simulink library "dynamics_lib"  (R2023b)
settings: Solver=VariableStepAuto  StartTime=0.0  StopTime=10.0  RelTol=1e-3
libraries: Raptor_lib x129, cstblocks x1, autolibshared x1
(part 1 of 2)
settings Model: Creator=serga  LastModifiedBy=serga
settings OptimizationCC: ReuseModelBlockBuffer=off

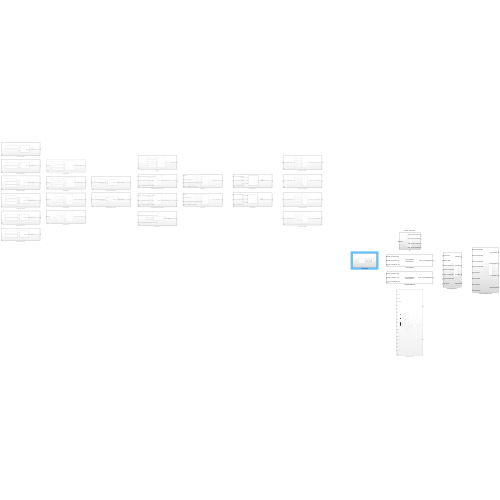
[thumbnail: Simulink's stored preview of the top-level diagram]
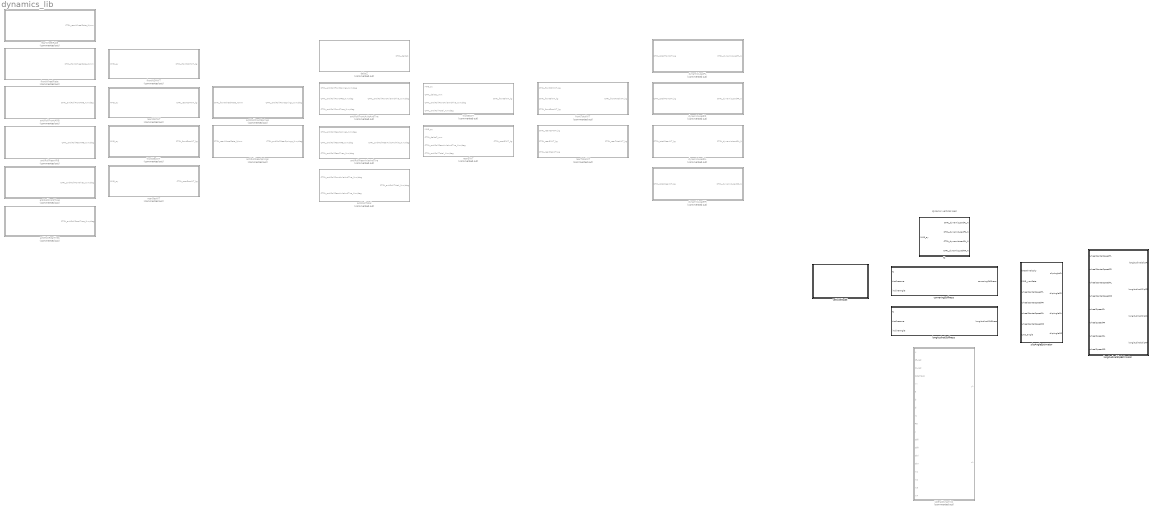
== system dynamics_lib ==
  note: dynamic vertical load
  antiRollFrontARB : Subsystem  Commented=on  TreatAsAtomicUnit=on
  antiRollFrontAxleAndTire : Subsystem  Commented=on  TreatAsAtomicUnit=on
  antiRollFrontSprings : Subsystem  Commented=on  TreatAsAtomicUnit=on
  antiRollFrontTires : Subsystem  Commented=on  TreatAsAtomicUnit=on
  antiRollRearARB : Subsystem  Commented=on  TreatAsAtomicUnit=on
  antiRollRearAxleAndTire : Subsystem  Commented=on  TreatAsAtomicUnit=on
  antiRollRearSprings : Subsystem  Commented=on  TreatAsAtomicUnit=on
  antiRollRearTires : Subsystem  Commented=on  TreatAsAtomicUnit=on
  antiRollTotal : Subsystem  Commented=on  TreatAsAtomicUnit=on
  corneringStiffness : Subsystem  mask{pos=''}
      mask Display:
      | disp(['corneringStiffness\n'...
      |     'Wheel Position: ' pos]);
      | port_label('input', 1, ['CTRL_dynamicLoad' pos '_N']);
      | port_label('input', 2, ['CTRL_tirePressure' pos '_bar']);
      | port_label('input', 3, ['CTRL_inclineAngle' pos '_deg']);
      | port_label('output', 1, ['CTRL_corneringStiffness' pos]);
  deltaZ : Subsystem  Commented=on  TreatAsAtomicUnit=on
  dynamicLoadFL : Subsystem  Commented=on  TreatAsAtomicUnit=on
  dynamicLoadFR : Subsystem  Commented=on  TreatAsAtomicUnit=on
  dynamicLoadRL : Subsystem  Commented=on  TreatAsAtomicUnit=on
  dynamicLoadRR : Subsystem  Commented=on  TreatAsAtomicUnit=on
  frontElWT : Subsystem  Commented=on  TreatAsAtomicUnit=on
  frontGeoWT : Subsystem  Commented=on  TreatAsAtomicUnit=on
  frontNSMWT : Subsystem  Commented=on
  frontTotalWT : Subsystem  Commented=on  TreatAsAtomicUnit=on
  frontWheelRate : Subsystem  Commented=on  TreatAsAtomicUnit=on
  fz : Subsystem
  lateralDynamics : Subsystem  Commented=on
  longitudinalSlipEstimator : Subsystem
  longitudinalStiffness : Subsystem  mask{pos=''}
      mask Display:
      | disp(['longitudinalStiffness\n'...
      |     'Wheel Position: ' pos]);
      | port_label('input', 1, ['CTRL_dynamicLoad' pos '_N']);
      | port_label('input', 2, ['CTRL_tirePressure' pos '_bar']);
      | port_label('input', 3, ['CTRL_inclineAngle' pos '_deg']);
      | port_label('output', 1, ['CTRL_longitudinalStiffness' pos]);
  rearElWT : Subsystem  Commented=on  TreatAsAtomicUnit=on
  rearGeoWT : Subsystem  Commented=on  TreatAsAtomicUnit=on
  rearNSMWT : Subsystem  Commented=on  TreatAsAtomicUnit=on
  rearTotalWT : Subsystem  Commented=on  TreatAsAtomicUnit=on
  rearWheelRate : Subsystem  Commented=on  TreatAsAtomicUnit=on
  slipAngleEstimator : Subsystem
  vehicleModel : Subsystem

== system dynamics_lib/antiRollFrontARB ==
  antiRollFrontARB : MATLAB Function  TreatAsAtomicUnit=on
  raptor_data_read : Raptor_lib/Data Storage/raptor_data_read  dataName='DATA_frontTrack_mm'  dataShape=Scalar  idxSource=Input  idxRow=1  idxCol=1
      settings: SourceProductName=Raptor
  raptor_data_read1 : Raptor_lib/Data Storage/raptor_data_read  dataName='DATA_frontARBStiffness_Npmm'  dataShape=Scalar  idxSource=Input  idxRow=1  idxCol=1
      settings: SourceProductName=Raptor
  raptor_data_read2 : Raptor_lib/Data Storage/raptor_data_read  dataName='DATA_frontARBMotionRatio_mmpmm'  dataShape=Scalar  idxSource=Input  idxRow=1  idxCol=1
      settings: SourceProductName=Raptor
  CTRL_antiRollFrontARB_N.m/deg : Outport
  wires:
  antiRollFrontARB/1(antiRollFrontARB) -> CTRL_antiRollFrontARB_N.m/deg/1
  raptor_data_read2/1 -> antiRollFrontARB/3(frontARBMotionRatio)
  raptor_data_read1/1 -> antiRollFrontARB/1(frontARBStiffness)
  raptor_data_read/1 -> antiRollFrontARB/2(frontTrack)

== system dynamics_lib/antiRollFrontAxleAndTire ==
  CTRL_antiRollFrontSprings_N.m/deg : Inport
  CTRL_antiRollFrontARB_N.m/deg : Inport  Port=2
  CTRL_antiRollFrontTires_N.m/deg : Inport  Port=3
  antiRollFrontAxleAndTire : MATLAB Function  TreatAsAtomicUnit=on
  CTRL_antiRollFrontAxleAndTire_N.m/deg : Outport
  wires:
  CTRL_antiRollFrontSprings_N.m/deg/1 -> antiRollFrontAxleAndTire/1(antiRollFrontSprings)
  CTRL_antiRollFrontARB_N.m/deg/1 -> antiRollFrontAxleAndTire/2(antiRollFrontARB)
  CTRL_antiRollFrontTires_N.m/deg/1 -> antiRollFrontAxleAndTire/3(antiRollFrontTires)
  antiRollFrontAxleAndTire/1(antiRollFrontAxleAndTire) -> CTRL_antiRollFrontAxleAndTire_N.m/deg/1

== system dynamics_lib/antiRollFrontSprings ==
  CTRL_frontWheelRate_N/mm : Inport
  antiRollFrontSprings : MATLAB Function  TreatAsAtomicUnit=on
  raptor_data_read : Raptor_lib/Data Storage/raptor_data_read  dataName='DATA_frontTrack_mm'  dataShape=Scalar  idxSource=Input  idxRow=1  idxCol=1
      settings: SourceProductName=Raptor
  CTRL_antiRollFrontSprings_N.m/deg : Outport
  wires:
  raptor_data_read/1 -> antiRollFrontSprings/1(frontTrack)
  CTRL_frontWheelRate_N/mm/1 -> antiRollFrontSprings/2(frontWheelRate)
  antiRollFrontSprings/1(antiRollFrontSprings) -> CTRL_antiRollFrontSprings_N.m/deg/1

== system dynamics_lib/antiRollFrontTires ==
  antiRollFrontTires : MATLAB Function  TreatAsAtomicUnit=on
  raptor_data_read : Raptor_lib/Data Storage/raptor_data_read  dataName='DATA_frontTrack_mm'  dataShape=Scalar  idxSource=Input  idxRow=1  idxCol=1
      settings: SourceProductName=Raptor
  raptor_data_read1 : Raptor_lib/Data Storage/raptor_data_read  dataName='DATA_frontTireStiffness_Npmm'  dataShape=Scalar  idxSource=Input  idxRow=1  idxCol=1
      settings: SourceProductName=Raptor
  CTRL_antiRollFrontTires_N.m/deg : Outport
  wires:
  raptor_data_read1/1 -> antiRollFrontTires/2(frontTireStiffness)
  raptor_data_read/1 -> antiRollFrontTires/1(frontTrack)
  antiRollFrontTires/1(antiRollFrontTires) -> CTRL_antiRollFrontTires_N.m/deg/1

== system dynamics_lib/antiRollRearARB ==
  antiRollRearARB : MATLAB Function  TreatAsAtomicUnit=on
  raptor_data_read : Raptor_lib/Data Storage/raptor_data_read  dataName='DATA_rearTrack_mm'  dataShape=Scalar  idxSource=Input  idxRow=1  idxCol=1
      settings: SourceProductName=Raptor
  raptor_data_read1 : Raptor_lib/Data Storage/raptor_data_read  dataName='DATA_rearARBStiffness_Npmm'  dataShape=Scalar  idxSource=Input  idxRow=1  idxCol=1
      settings: SourceProductName=Raptor
  raptor_data_read2 : Raptor_lib/Data Storage/raptor_data_read  dataName='DATA_rearARBMotionRatio_mmpmm'  dataShape=Scalar  idxSource=Input  idxRow=1  idxCol=1
      settings: SourceProductName=Raptor
  CTRL_antiRollRearARB_N.m/deg : Outport
  wires:
  raptor_data_read2/1 -> antiRollRearARB/3(rearARBMotionRatio)
  raptor_data_read1/1 -> antiRollRearARB/1(rearARBStiffness)
  raptor_data_read/1 -> antiRollRearARB/2(rearTrack)
  antiRollRearARB/1(antiRollRearARB) -> CTRL_antiRollRearARB_N.m/deg/1

== system dynamics_lib/antiRollRearAxleAndTire ==
  CTRL_antiRollRearSprings_N.m/deg : Inport
  CTRL_antiRollRearARB_N.m/deg : Inport  Port=2
  CTRL_antiRollRearTires_N.m/deg : Inport  Port=3
  antiRollRearAxleAndTire : MATLAB Function  TreatAsAtomicUnit=on
  CTRL_antiRollRearAxleAndTire_N.m/deg : Outport
  wires:
  CTRL_antiRollRearSprings_N.m/deg/1 -> antiRollRearAxleAndTire/1(antiRollRearSprings)
  CTRL_antiRollRearARB_N.m/deg/1 -> antiRollRearAxleAndTire/2(antiRollRearARB)
  CTRL_antiRollRearTires_N.m/deg/1 -> antiRollRearAxleAndTire/3(antiRollRearTires)
  antiRollRearAxleAndTire/1(antiRollRearAxleAndTire) -> CTRL_antiRollRearAxleAndTire_N.m/deg/1

== system dynamics_lib/antiRollRearSprings ==
  CTRL_rearWheelRate_N/mm : Inport
  antiRollRearSprings : MATLAB Function  TreatAsAtomicUnit=on
  raptor_data_read : Raptor_lib/Data Storage/raptor_data_read  dataName='DATA_rearTrack_mm'  dataShape=Scalar  idxSource=Input  idxRow=1  idxCol=1
      settings: SourceProductName=Raptor
  CTRL_antiRollRearSprings_N.m/deg : Outport
  wires:
  raptor_data_read/1 -> antiRollRearSprings/1(rearTrack)
  CTRL_rearWheelRate_N/mm/1 -> antiRollRearSprings/2(rearWheelRate)
  antiRollRearSprings/1(antiRollRearSprings) -> CTRL_antiRollRearSprings_N.m/deg/1

== system dynamics_lib/antiRollRearTires ==
  antiRollRearTires : MATLAB Function  TreatAsAtomicUnit=on
  raptor_data_read : Raptor_lib/Data Storage/raptor_data_read  dataName='DATA_rearTrack_mm'  dataShape=Scalar  idxSource=Input  idxRow=1  idxCol=1
      settings: SourceProductName=Raptor
  raptor_data_read1 : Raptor_lib/Data Storage/raptor_data_read  dataName='DATA_rearTireStiffness_Npmm'  dataShape=Scalar  idxSource=Input  idxRow=1  idxCol=1
      settings: SourceProductName=Raptor
  CTRL_antiRollRearTires_N.m/deg : Outport
  wires:
  raptor_data_read1/1 -> antiRollRearTires/2(rearTireStiffness)
  raptor_data_read/1 -> antiRollRearTires/1(rearTrack)
  antiRollRearTires/1(antiRollRearTires) -> CTRL_antiRollRearTires_N.m/deg/1

== system dynamics_lib/antiRollTotal ==
  CTRL_antiRollFrontAxleAndTire_N.m/deg : Inport
  CTRL_antiRollRearAxleAndTire_N.m/deg : Inport  Port=2
  antiRollTotal : MATLAB Function  TreatAsAtomicUnit=on
  CTRL_antiRollTotal_N.m/deg : Outport
  wires:
  antiRollTotal/1(antiRollTotal) -> CTRL_antiRollTotal_N.m/deg/1
  CTRL_antiRollFrontAxleAndTire_N.m/deg/1 -> antiRollTotal/1(antiRollFrontAxleAndTire)
  CTRL_antiRollRearAxleAndTire_N.m/deg/1 -> antiRollTotal/2(antiRollRearAxleAndTire)

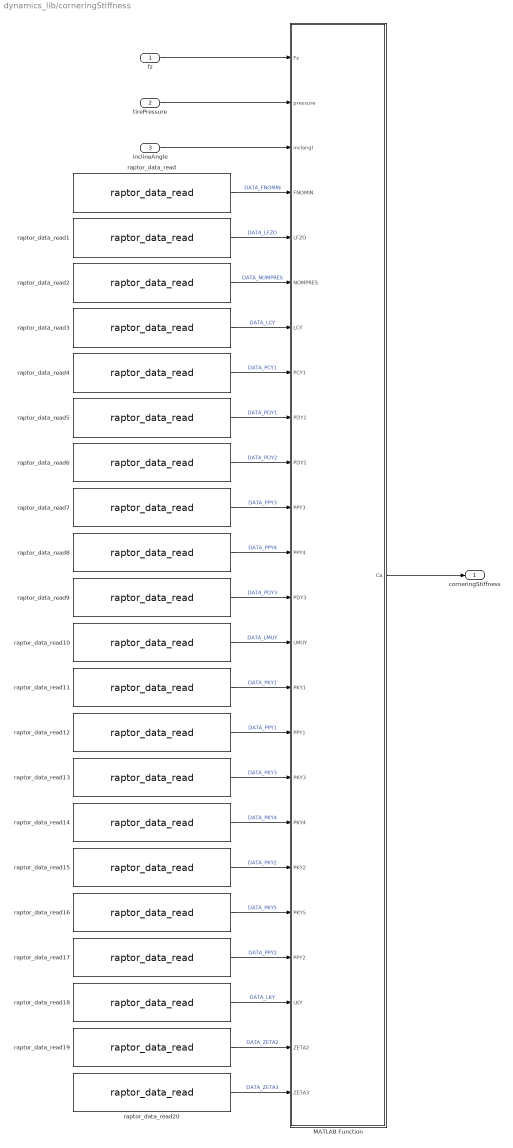
== system dynamics_lib/corneringStiffness ==
  fz : Inport
  tirePressure : Inport  Port=2
  inclineAngle : Inport  Port=3
  MATLAB Function : MATLAB Function  TreatAsAtomicUnit=on
  raptor_data_read : Raptor_lib/Data Storage/raptor_data_read  dataName='DATA_FNOMIN_CS'  dataShape=Scalar  idxSource=Input  idxRow=1  idxCol=1
      settings: SourceProductName=Raptor
  raptor_data_read1 : Raptor_lib/Data Storage/raptor_data_read  dataName='DATA_LFZO'  dataShape=Scalar  idxSource=Input  idxRow=1  idxCol=1
      settings: SourceProductName=Raptor
  raptor_data_read10 : Raptor_lib/Data Storage/raptor_data_read  dataName='DATA_LMUY'  dataShape=Scalar  idxSource=Input  idxRow=1  idxCol=1
      settings: SourceProductName=Raptor
  raptor_data_read11 : Raptor_lib/Data Storage/raptor_data_read  dataName='DATA_PKY1'  dataShape=Scalar  idxSource=Input  idxRow=1  idxCol=1
      settings: SourceProductName=Raptor
  raptor_data_read12 : Raptor_lib/Data Storage/raptor_data_read  dataName='DATA_PPY1'  dataShape=Scalar  idxSource=Input  idxRow=1  idxCol=1
      settings: SourceProductName=Raptor
  raptor_data_read13 : Raptor_lib/Data Storage/raptor_data_read  dataName='DATA_PKY3'  dataShape=Scalar  idxSource=Input  idxRow=1  idxCol=1
      settings: SourceProductName=Raptor
  raptor_data_read14 : Raptor_lib/Data Storage/raptor_data_read  dataName='DATA_PKY4'  dataShape=Scalar  idxSource=Input  idxRow=1  idxCol=1
      settings: SourceProductName=Raptor
  raptor_data_read15 : Raptor_lib/Data Storage/raptor_data_read  dataName='DATA_PKY2'  dataShape=Scalar  idxSource=Input  idxRow=1  idxCol=1
      settings: SourceProductName=Raptor
  raptor_data_read16 : Raptor_lib/Data Storage/raptor_data_read  dataName='DATA_PKY5'  dataShape=Scalar  idxSource=Input  idxRow=1  idxCol=1
      settings: SourceProductName=Raptor
  raptor_data_read17 : Raptor_lib/Data Storage/raptor_data_read  dataName='DATA_PPY2'  dataShape=Scalar  idxSource=Input  idxRow=1  idxCol=1
      settings: SourceProductName=Raptor
  raptor_data_read18 : Raptor_lib/Data Storage/raptor_data_read  dataName='DATA_LKY'  dataShape=Scalar  idxSource=Input  idxRow=1  idxCol=1
      settings: SourceProductName=Raptor
  raptor_data_read19 : Raptor_lib/Data Storage/raptor_data_read  dataName='DATA_ZETA2'  dataShape=Scalar  idxSource=Input  idxRow=1  idxCol=1
      settings: SourceProductName=Raptor
  raptor_data_read2 : Raptor_lib/Data Storage/raptor_data_read  dataName='DATA_NOMPRES_CS'  dataShape=Scalar  idxSource=Input  idxRow=1  idxCol=1
      settings: SourceProductName=Raptor
  raptor_data_read20 : Raptor_lib/Data Storage/raptor_data_read  dataName='DATA_ZETA3'  dataShape=Scalar  idxSource=Input  idxRow=1  idxCol=1
      settings: SourceProductName=Raptor
  raptor_data_read3 : Raptor_lib/Data Storage/raptor_data_read  dataName='DATA_LCY'  dataShape=Scalar  idxSource=Input  idxRow=1  idxCol=1
      settings: SourceProductName=Raptor
  raptor_data_read4 : Raptor_lib/Data Storage/raptor_data_read  dataName='DATA_PCY1'  dataShape=Scalar  idxSource=Input  idxRow=1  idxCol=1
      settings: SourceProductName=Raptor
  raptor_data_read5 : Raptor_lib/Data Storage/raptor_data_read  dataName='DATA_PDY1'  dataShape=Scalar  idxSource=Input  idxRow=1  idxCol=1
      settings: SourceProductName=Raptor
  raptor_data_read6 : Raptor_lib/Data Storage/raptor_data_read  dataName='DATA_PDY2'  dataShape=Scalar  idxSource=Input  idxRow=1  idxCol=1
      settings: SourceProductName=Raptor
  raptor_data_read7 : Raptor_lib/Data Storage/raptor_data_read  dataName='DATA_PPY3'  dataShape=Scalar  idxSource=Input  idxRow=1  idxCol=1
      settings: SourceProductName=Raptor
  raptor_data_read8 : Raptor_lib/Data Storage/raptor_data_read  dataName='DATA_PPY4'  dataShape=Scalar  idxSource=Input  idxRow=1  idxCol=1
      settings: SourceProductName=Raptor
  raptor_data_read9 : Raptor_lib/Data Storage/raptor_data_read  dataName='DATA_PDY3'  dataShape=Scalar  idxSource=Input  idxRow=1  idxCol=1
      settings: SourceProductName=Raptor
  corneringStiffness : Outport
  wires:
  raptor_data_read20/1 -> MATLAB Function/24(ZETA3)  "DATA_ZETA3"
  raptor_data_read19/1 -> MATLAB Function/23(ZETA2)  "DATA_ZETA2"
  raptor_data_read18/1 -> MATLAB Function/22(LKY)  "DATA_LKY"
  raptor_data_read17/1 -> MATLAB Function/21(PPY2)  "DATA_PPY2"
  raptor_data_read16/1 -> MATLAB Function/20(PKY5)  "DATA_PKY5"
  raptor_data_read15/1 -> MATLAB Function/19(PKY2)  "DATA_PKY2"
  raptor_data_read14/1 -> MATLAB Function/18(PKY4)  "DATA_PKY4"
  raptor_data_read13/1 -> MATLAB Function/17(PKY3)  "DATA_PKY3"
  raptor_data_read12/1 -> MATLAB Function/16(PPY1)  "DATA_PPY1"
  raptor_data_read11/1 -> MATLAB Function/15(PKY1)  "DATA_PKY1"
  raptor_data_read10/1 -> MATLAB Function/14(LMUY)  "DATA_LMUY"
  raptor_data_read9/1 -> MATLAB Function/13(PDY3)  "DATA_PDY3"
  raptor_data_read8/1 -> MATLAB Function/12(PPY4)  "DATA_PPY4"
  raptor_data_read7/1 -> MATLAB Function/11(PPY3)  "DATA_PPY3"
  raptor_data_read6/1 -> MATLAB Function/10(PDY2)  "DATA_PDY2"
  raptor_data_read5/1 -> MATLAB Function/9(PDY1)  "DATA_PDY1"
  raptor_data_read4/1 -> MATLAB Function/8(PCY1)  "DATA_PCY1"
  raptor_data_read3/1 -> MATLAB Function/7(LCY)  "DATA_LCY"
  raptor_data_read2/1 -> MATLAB Function/6(NOMPRES)  "DATA_NOMPRES"
  raptor_data_read1/1 -> MATLAB Function/5(LFZO)  "DATA_LFZO"
  raptor_data_read/1 -> MATLAB Function/4(FNOMIN)  "DATA_FNOMIN"
  inclineAngle/1 -> MATLAB Function/3(inclangl)
  fz/1 -> MATLAB Function/1(Fz)
  tirePressure/1 -> MATLAB Function/2(pressure)
  MATLAB Function/1(Ca) -> corneringStiffness/1

== system dynamics_lib/deltaZ ==
  deltaZ : MATLAB Function  TreatAsAtomicUnit=on
  raptor_data_read : Raptor_lib/Data Storage/raptor_data_read  dataName='DATA_wheelBase_mm'  dataShape=Scalar  idxSource=Input  idxRow=1  idxCol=1
      settings: SourceProductName=Raptor
  raptor_data_read1 : Raptor_lib/Data Storage/raptor_data_read  dataName='DATA_suspendedMassWeightDistribution_pct'  dataShape=Scalar  idxSource=Input  idxRow=1  idxCol=1
      settings: SourceProductName=Raptor
  raptor_data_read2 : Raptor_lib/Data Storage/raptor_data_read  dataName='DATA_suspendedMassCGCoordinatesZ_mm'  dataShape=Scalar  idxSource=Input  idxRow=1  idxCol=1
      settings: SourceProductName=Raptor
  raptor_data_read3 : Raptor_lib/Data Storage/raptor_data_read  dataName='DATA_frontRollCenterHeight_mm'  dataShape=Scalar  idxSource=Input  idxRow=1  idxCol=1
      settings: SourceProductName=Raptor
  raptor_data_read4 : Raptor_lib/Data Storage/raptor_data_read  dataName='DATA_rearRollCenterHeight_mm'  dataShape=Scalar  idxSource=Input  idxRow=1  idxCol=1
      settings: SourceProductName=Raptor
  CTRL_deltaZ : Outport
  wires:
  raptor_data_read1/1 -> deltaZ/2(suspendedMassWeightDistribution)
  raptor_data_read/1 -> deltaZ/1(wheelBase)
  raptor_data_read3/1 -> deltaZ/4(frontRollCenterHeight)
  raptor_data_read4/1 -> deltaZ/5(rearRollCenterHeight)
  raptor_data_read2/1 -> deltaZ/3(suspendedMassCGCoordinatesZ)
  deltaZ/1(deltaZ) -> CTRL_deltaZ/1

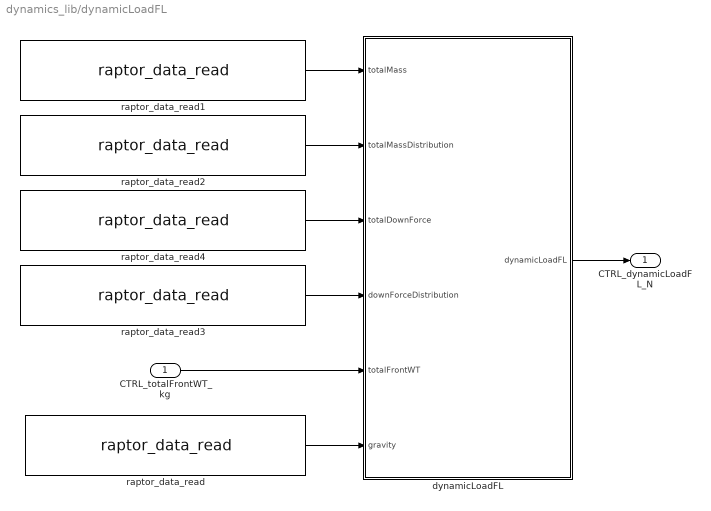
== system dynamics_lib/dynamicLoadFL ==
  CTRL_totalFrontWT_kg : Inport
  dynamicLoadFL : MATLAB Function  TreatAsAtomicUnit=on
  raptor_data_read : Raptor_lib/Data Storage/raptor_data_read  dataName='DATA_gravity_mpsec2'  dataShape=Scalar  idxSource=Input  idxRow=1  idxCol=1
      settings: SourceProductName=Raptor
  raptor_data_read1 : Raptor_lib/Data Storage/raptor_data_read  dataName='DATA_totalMass_kg'  dataShape=Scalar  idxSource=Input  idxRow=1  idxCol=1
      settings: SourceProductName=Raptor
  raptor_data_read2 : Raptor_lib/Data Storage/raptor_data_read  dataName='DATA_totalMassDistribution_pct'  dataShape=Scalar  idxSource=Input  idxRow=1  idxCol=1
      settings: SourceProductName=Raptor
  raptor_data_read3 : Raptor_lib/Data Storage/raptor_data_read  dataName='DATA_downForceDistribution_pct'  dataShape=Scalar  idxSource=Input  idxRow=1  idxCol=1
      settings: SourceProductName=Raptor
  raptor_data_read4 : Raptor_lib/Data Storage/raptor_data_read  dataName='DATA_totalDownForce_kg'  dataShape=Scalar  idxSource=Input  idxRow=1  idxCol=1
      settings: SourceProductName=Raptor
  CTRL_dynamicLoadFL_N : Outport
  wires:
  raptor_data_read1/1 -> dynamicLoadFL/1(totalMass)
  raptor_data_read2/1 -> dynamicLoadFL/2(totalMassDistribution)
  raptor_data_read4/1 -> dynamicLoadFL/3(totalDownForce)
  raptor_data_read3/1 -> dynamicLoadFL/4(downForceDistribution)
  CTRL_totalFrontWT_kg/1 -> dynamicLoadFL/5(totalFrontWT)
  raptor_data_read/1 -> dynamicLoadFL/6(gravity)
  dynamicLoadFL/1(dynamicLoadFL) -> CTRL_dynamicLoadFL_N/1

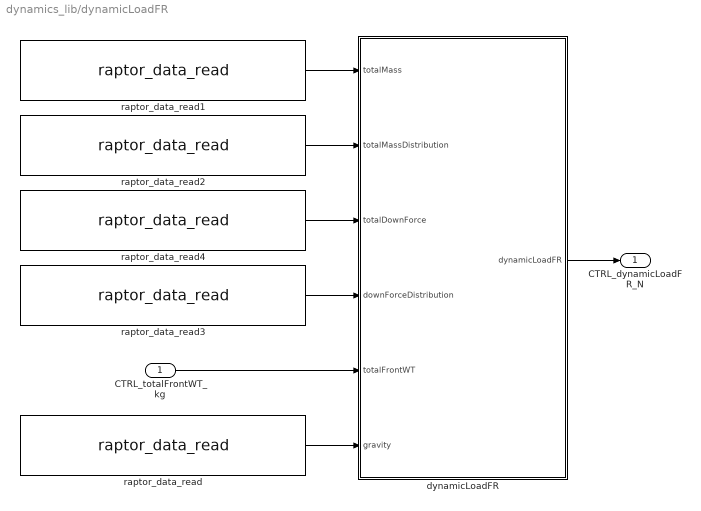
== system dynamics_lib/dynamicLoadFR ==
  CTRL_totalFrontWT_kg : Inport
  dynamicLoadFR : MATLAB Function  TreatAsAtomicUnit=on
  raptor_data_read : Raptor_lib/Data Storage/raptor_data_read  dataName='DATA_gravity_mpsec2'  dataShape=Scalar  idxSource=Input  idxRow=1  idxCol=1
      settings: SourceProductName=Raptor
  raptor_data_read1 : Raptor_lib/Data Storage/raptor_data_read  dataName='DATA_totalMass_kg'  dataShape=Scalar  idxSource=Input  idxRow=1  idxCol=1
      settings: SourceProductName=Raptor
  raptor_data_read2 : Raptor_lib/Data Storage/raptor_data_read  dataName='DATA_totalMassDistribution_pct'  dataShape=Scalar  idxSource=Input  idxRow=1  idxCol=1
      settings: SourceProductName=Raptor
  raptor_data_read3 : Raptor_lib/Data Storage/raptor_data_read  dataName='DATA_downForceDistribution_pct'  dataShape=Scalar  idxSource=Input  idxRow=1  idxCol=1
      settings: SourceProductName=Raptor
  raptor_data_read4 : Raptor_lib/Data Storage/raptor_data_read  dataName='DATA_totalDownForce_kg'  dataShape=Scalar  idxSource=Input  idxRow=1  idxCol=1
      settings: SourceProductName=Raptor
  CTRL_dynamicLoadFR_N : Outport
  wires:
  raptor_data_read1/1 -> dynamicLoadFR/1(totalMass)
  raptor_data_read2/1 -> dynamicLoadFR/2(totalMassDistribution)
  raptor_data_read4/1 -> dynamicLoadFR/3(totalDownForce)
  raptor_data_read3/1 -> dynamicLoadFR/4(downForceDistribution)
  CTRL_totalFrontWT_kg/1 -> dynamicLoadFR/5(totalFrontWT)
  raptor_data_read/1 -> dynamicLoadFR/6(gravity)
  dynamicLoadFR/1(dynamicLoadFR) -> CTRL_dynamicLoadFR_N/1

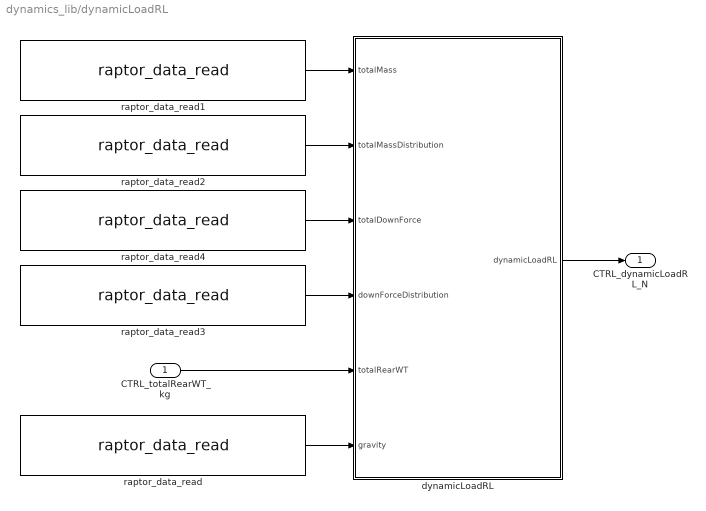
== system dynamics_lib/dynamicLoadRL ==
  CTRL_totalRearWT_kg : Inport
  dynamicLoadRL : MATLAB Function  TreatAsAtomicUnit=on
  raptor_data_read : Raptor_lib/Data Storage/raptor_data_read  dataName='DATA_gravity_mpsec2'  dataShape=Scalar  idxSource=Input  idxRow=1  idxCol=1
      settings: SourceProductName=Raptor
  raptor_data_read1 : Raptor_lib/Data Storage/raptor_data_read  dataName='DATA_totalMass_kg'  dataShape=Scalar  idxSource=Input  idxRow=1  idxCol=1
      settings: SourceProductName=Raptor
  raptor_data_read2 : Raptor_lib/Data Storage/raptor_data_read  dataName='DATA_totalMassDistribution_pct'  dataShape=Scalar  idxSource=Input  idxRow=1  idxCol=1
      settings: SourceProductName=Raptor
  raptor_data_read3 : Raptor_lib/Data Storage/raptor_data_read  dataName='DATA_downForceDistribution_pct'  dataShape=Scalar  idxSource=Input  idxRow=1  idxCol=1
      settings: SourceProductName=Raptor
  raptor_data_read4 : Raptor_lib/Data Storage/raptor_data_read  dataName='DATA_totalDownForce_kg'  dataShape=Scalar  idxSource=Input  idxRow=1  idxCol=1
      settings: SourceProductName=Raptor
  CTRL_dynamicLoadRL_N : Outport
  wires:
  raptor_data_read1/1 -> dynamicLoadRL/1(totalMass)
  raptor_data_read2/1 -> dynamicLoadRL/2(totalMassDistribution)
  raptor_data_read4/1 -> dynamicLoadRL/3(totalDownForce)
  raptor_data_read3/1 -> dynamicLoadRL/4(downForceDistribution)
  CTRL_totalRearWT_kg/1 -> dynamicLoadRL/5(totalRearWT)
  raptor_data_read/1 -> dynamicLoadRL/6(gravity)
  dynamicLoadRL/1(dynamicLoadRL) -> CTRL_dynamicLoadRL_N/1

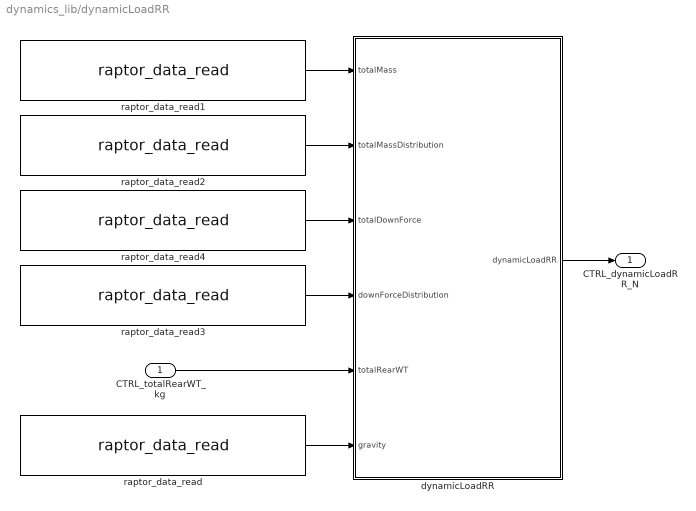
== system dynamics_lib/dynamicLoadRR ==
  CTRL_totalRearWT_kg : Inport
  dynamicLoadRR : MATLAB Function  TreatAsAtomicUnit=on
  raptor_data_read : Raptor_lib/Data Storage/raptor_data_read  dataName='DATA_gravity_mpsec2'  dataShape=Scalar  idxSource=Input  idxRow=1  idxCol=1
      settings: SourceProductName=Raptor
  raptor_data_read1 : Raptor_lib/Data Storage/raptor_data_read  dataName='DATA_totalMass_kg'  dataShape=Scalar  idxSource=Input  idxRow=1  idxCol=1
      settings: SourceProductName=Raptor
  raptor_data_read2 : Raptor_lib/Data Storage/raptor_data_read  dataName='DATA_totalMassDistribution_pct'  dataShape=Scalar  idxSource=Input  idxRow=1  idxCol=1
      settings: SourceProductName=Raptor
  raptor_data_read3 : Raptor_lib/Data Storage/raptor_data_read  dataName='DATA_downForceDistribution_pct'  dataShape=Scalar  idxSource=Input  idxRow=1  idxCol=1
      settings: SourceProductName=Raptor
  raptor_data_read4 : Raptor_lib/Data Storage/raptor_data_read  dataName='DATA_totalDownForce_kg'  dataShape=Scalar  idxSource=Input  idxRow=1  idxCol=1
      settings: SourceProductName=Raptor
  CTRL_dynamicLoadRR_N : Outport
  wires:
  raptor_data_read1/1 -> dynamicLoadRR/1(totalMass)
  raptor_data_read2/1 -> dynamicLoadRR/2(totalMassDistribution)
  raptor_data_read4/1 -> dynamicLoadRR/3(totalDownForce)
  raptor_data_read3/1 -> dynamicLoadRR/4(downForceDistribution)
  CTRL_totalRearWT_kg/1 -> dynamicLoadRR/5(totalRearWT)
  raptor_data_read/1 -> dynamicLoadRR/6(gravity)
  dynamicLoadRR/1(dynamicLoadRR) -> CTRL_dynamicLoadRR_N/1

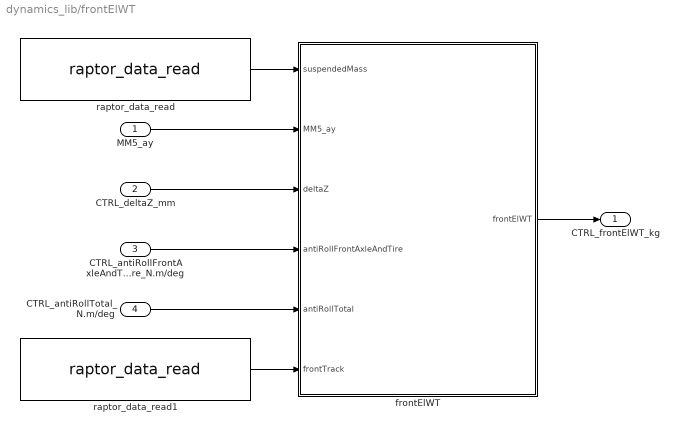
== system dynamics_lib/frontElWT ==
  MM5_ay : Inport
  CTRL_deltaZ_mm : Inport  Port=2
  CTRL_antiRollFrontAxleAndTire_N.m/deg : Inport  Port=3
  CTRL_antiRollTotal_N.m/deg : Inport  Port=4
  frontElWT : MATLAB Function  TreatAsAtomicUnit=on
  raptor_data_read : Raptor_lib/Data Storage/raptor_data_read  dataName='DATA_suspendedMass_kg'  dataShape=Scalar  idxSource=Input  idxRow=1  idxCol=1
      settings: SourceProductName=Raptor
  raptor_data_read1 : Raptor_lib/Data Storage/raptor_data_read  dataName='DATA_frontTrack_mm'  dataShape=Scalar  idxSource=Input  idxRow=1  idxCol=1
      settings: SourceProductName=Raptor
  CTRL_frontElWT_kg : Outport
  wires:
  raptor_data_read/1 -> frontElWT/1(suspendedMass)
  MM5_ay/1 -> frontElWT/2(MM5_ay)
  CTRL_deltaZ_mm/1 -> frontElWT/3(deltaZ)
  raptor_data_read1/1 -> frontElWT/6(frontTrack)
  CTRL_antiRollFrontAxleAndTire_N.m/deg/1 -> frontElWT/4(antiRollFrontAxleAndTire)
  CTRL_antiRollTotal_N.m/deg/1 -> frontElWT/5(antiRollTotal)
  frontElWT/1(frontElWT) -> CTRL_frontElWT_kg/1

== system dynamics_lib/frontGeoWT ==
  MM5_ay : Inport
  frontGeoWT : MATLAB Function  TreatAsAtomicUnit=on
  raptor_data_read : Raptor_lib/Data Storage/raptor_data_read  dataName='DATA_suspendedMass_kg'  dataShape=Scalar  idxSource=Input  idxRow=1  idxCol=1
      settings: SourceProductName=Raptor
  raptor_data_read1 : Raptor_lib/Data Storage/raptor_data_read  dataName='DATA_suspendedMassWeightDistribution_pct'  dataShape=Scalar  idxSource=Input  idxRow=1  idxCol=1
      settings: SourceProductName=Raptor
  raptor_data_read2 : Raptor_lib/Data Storage/raptor_data_read  dataName='DATA_frontTrack_mm'  dataShape=Scalar  idxSource=Input  idxRow=1  idxCol=1
      settings: SourceProductName=Raptor
  raptor_data_read3 : Raptor_lib/Data Storage/raptor_data_read  dataName='DATA_frontRollCenterHeight_mm'  dataShape=Scalar  idxSource=Input  idxRow=1  idxCol=1
      settings: SourceProductName=Raptor
  CTRL_frontGeoWT_kg : Outport
  wires:
  raptor_data_read1/1 -> frontGeoWT/2(suspendedMassWeightDistribution)
  raptor_data_read/1 -> frontGeoWT/1(suspendedMass)
  MM5_ay/1 -> frontGeoWT/3(MM5_ay)
  raptor_data_read2/1 -> frontGeoWT/5(frontTrack)
  raptor_data_read3/1 -> frontGeoWT/4(frontRollCenterHeight)
  frontGeoWT/1(frontGeoWT) -> CTRL_frontGeoWT_kg/1

== system dynamics_lib/frontNSMWT ==
  MM5_ay : Inport
  frontNSMWT : MATLAB Function  TreatAsAtomicUnit=on
  raptor_data_read : Raptor_lib/Data Storage/raptor_data_read  dataName='DATA_frontNonSuspendedMass_kg'  dataShape=Scalar  idxSource=Input  idxRow=1  idxCol=1
      settings: SourceProductName=Raptor
  raptor_data_read1 : Raptor_lib/Data Storage/raptor_data_read  dataName='DATA_frontNonSuspendedMassCGHeight_mm'  dataShape=Scalar  idxSource=Input  idxRow=1  idxCol=1
      settings: SourceProductName=Raptor
  raptor_data_read2 : Raptor_lib/Data Storage/raptor_data_read  dataName='DATA_frontTrack_mm'  dataShape=Scalar  idxSource=Input  idxRow=1  idxCol=1
      settings: SourceProductName=Raptor
  CTRL_frontNSMWT_kg : Outport
  wires:
  frontNSMWT/1(frontNSMWT) -> CTRL_frontNSMWT_kg/1
  raptor_data_read2/1 -> frontNSMWT/4(frontTrack)
  raptor_data_read1/1 -> frontNSMWT/3(frontNonSuspendedMassCGHeight)
  MM5_ay/1 -> frontNSMWT/2(MM5_ay)
  raptor_data_read/1 -> frontNSMWT/1(frontNonSuspendedMass)

== system dynamics_lib/frontTotalWT ==
  CTRL_frontNSMWT_kg : Inport
  CTRL_frontElWT_kg : Inport  Port=2
  CTRL_frontGeoWT_kg : Inport  Port=3
  frontTotalWT : MATLAB Function  TreatAsAtomicUnit=on
  CTRL_frontTotalWT_kg : Outport
  wires:
  frontTotalWT/1(frontTotalWT) -> CTRL_frontTotalWT_kg/1
  CTRL_frontNSMWT_kg/1 -> frontTotalWT/1(frontNSMWT)
  CTRL_frontElWT_kg/1 -> frontTotalWT/2(frontElWT)
  CTRL_frontGeoWT_kg/1 -> frontTotalWT/3(frontGeoWT)

== system dynamics_lib/frontWheelRate ==
  frontWheelRate : MATLAB Function  TreatAsAtomicUnit=on
  raptor_data_read : Raptor_lib/Data Storage/raptor_data_read  dataName='DATA_frontSpringStiffness_Npmm'  dataShape=Scalar  idxSource=Input  idxRow=1  idxCol=1
      settings: SourceProductName=Raptor
  raptor_data_read2 : Raptor_lib/Data Storage/raptor_data_read  dataName='DATA_frontSpringMotionRatio_mmpmm'  dataShape=Scalar  idxSource=Input  idxRow=1  idxCol=1
      settings: SourceProductName=Raptor
  CTRL_frontWheelRate_N/mm : Outport
  wires:
  raptor_data_read2/1 -> frontWheelRate/2(frontSpringMotionRatio)
  raptor_data_read/1 -> frontWheelRate/1(frontSpringStiffness)
  frontWheelRate/1(frontWheelRate) -> CTRL_frontWheelRate_N/mm/1

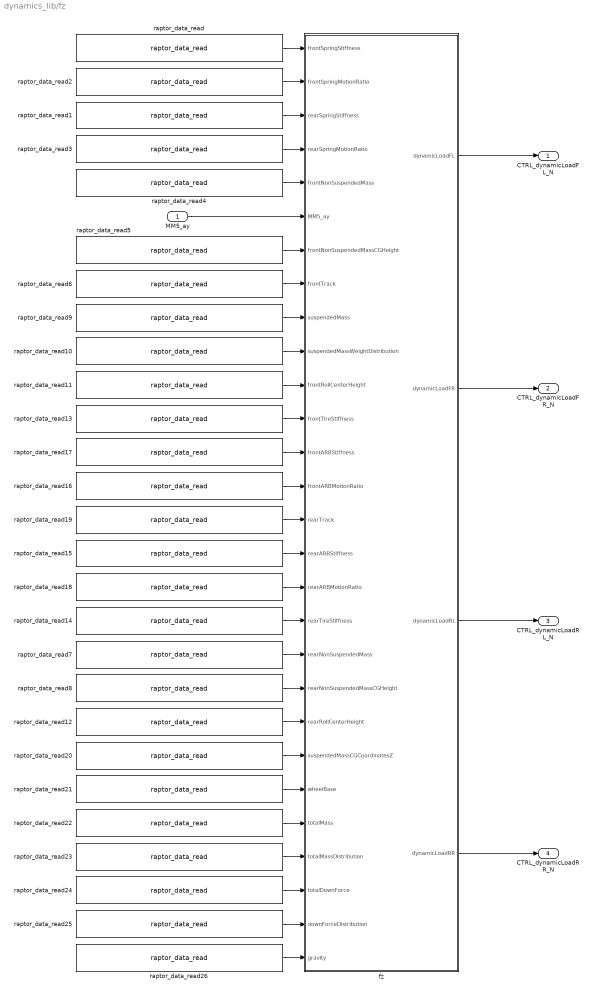
== system dynamics_lib/fz ==
  MM5_ay : Inport
  fz : MATLAB Function  TreatAsAtomicUnit=on
  raptor_data_read : Raptor_lib/Data Storage/raptor_data_read  dataName='DATA_frontSpringStiffness_Npmm'  dataShape=Scalar  idxSource=Input  idxRow=1  idxCol=1
      settings: SourceProductName=Raptor
  raptor_data_read1 : Raptor_lib/Data Storage/raptor_data_read  dataName='DATA_rearSpringStiffness_Npmm'  dataShape=Scalar  idxSource=Input  idxRow=1  idxCol=1
      settings: SourceProductName=Raptor
  raptor_data_read10 : Raptor_lib/Data Storage/raptor_data_read  dataName='DATA_suspendedMassWeightDistribution_pct'  dataShape=Scalar  idxSource=Input  idxRow=1  idxCol=1
      settings: SourceProductName=Raptor
  raptor_data_read11 : Raptor_lib/Data Storage/raptor_data_read  dataName='DATA_frontRollCenterHeight_mm'  dataShape=Scalar  idxSource=Input  idxRow=1  idxCol=1
      settings: SourceProductName=Raptor
  raptor_data_read12 : Raptor_lib/Data Storage/raptor_data_read  dataName='DATA_rearRollCenterHeight_mm'  dataShape=Scalar  idxSource=Input  idxRow=1  idxCol=1
      settings: SourceProductName=Raptor
  raptor_data_read13 : Raptor_lib/Data Storage/raptor_data_read  dataName='DATA_frontTireStiffness_Npmm'  dataShape=Scalar  idxSource=Input  idxRow=1  idxCol=1
      settings: SourceProductName=Raptor
  raptor_data_read14 : Raptor_lib/Data Storage/raptor_data_read  dataName='DATA_rearTireStiffness_Npmm'  dataShape=Scalar  idxSource=Input  idxRow=1  idxCol=1
      settings: SourceProductName=Raptor
  raptor_data_read15 : Raptor_lib/Data Storage/raptor_data_read  dataName='DATA_rearARBStiffness_Npmm'  dataShape=Scalar  idxSource=Input  idxRow=1  idxCol=1
      settings: SourceProductName=Raptor
  raptor_data_read16 : Raptor_lib/Data Storage/raptor_data_read  dataName='DATA_frontARBMotionRatio_mmpmm'  dataShape=Scalar  idxSource=Input  idxRow=1  idxCol=1
      settings: SourceProductName=Raptor
  raptor_data_read17 : Raptor_lib/Data Storage/raptor_data_read  dataName='DATA_frontARBStiffness_Npmm'  dataShape=Scalar  idxSource=Input  idxRow=1  idxCol=1
      settings: SourceProductName=Raptor
  raptor_data_read18 : Raptor_lib/Data Storage/raptor_data_read  dataName='DATA_rearARBMotionRatio_mmpmm'  dataShape=Scalar  idxSource=Input  idxRow=1  idxCol=1
      settings: SourceProductName=Raptor
  raptor_data_read19 : Raptor_lib/Data Storage/raptor_data_read  dataName='DATA_rearTrack_mm'  dataShape=Scalar  idxSource=Input  idxRow=1  idxCol=1
      settings: SourceProductName=Raptor
  raptor_data_read2 : Raptor_lib/Data Storage/raptor_data_read  dataName='DATA_frontSpringMotionRatio_mmpmm'  dataShape=Scalar  idxSource=Input  idxRow=1  idxCol=1
      settings: SourceProductName=Raptor
  raptor_data_read20 : Raptor_lib/Data Storage/raptor_data_read  dataName='DATA_suspendedMassCGCoordinatesZ_mm'  dataShape=Scalar  idxSource=Input  idxRow=1  idxCol=1
      settings: SourceProductName=Raptor
  raptor_data_read21 : Raptor_lib/Data Storage/raptor_data_read  dataName='DATA_wheelBase_mm'  dataShape=Scalar  idxSource=Input  idxRow=1  idxCol=1
      settings: SourceProductName=Raptor
  raptor_data_read22 : Raptor_lib/Data Storage/raptor_data_read  dataName='DATA_totalMass_kg'  dataShape=Scalar  idxSource=Input  idxRow=1  idxCol=1
      settings: SourceProductName=Raptor
  raptor_data_read23 : Raptor_lib/Data Storage/raptor_data_read  dataName='DATA_totalMassDistribution_pct'  dataShape=Scalar  idxSource=Input  idxRow=1  idxCol=1
      settings: SourceProductName=Raptor
  raptor_data_read24 : Raptor_lib/Data Storage/raptor_data_read  dataName='DATA_totalDownForce_kg'  dataShape=Scalar  idxSource=Input  idxRow=1  idxCol=1
      settings: SourceProductName=Raptor
  raptor_data_read25 : Raptor_lib/Data Storage/raptor_data_read  dataName='DATA_downForceDistribution_pct'  dataShape=Scalar  idxSource=Input  idxRow=1  idxCol=1
      settings: SourceProductName=Raptor
  raptor_data_read26 : Raptor_lib/Data Storage/raptor_data_read  dataName='DATA_gravity_mpsec2'  dataShape=Scalar  idxSource=Input  idxRow=1  idxCol=1
      settings: SourceProductName=Raptor
  raptor_data_read3 : Raptor_lib/Data Storage/raptor_data_read  dataName='DATA_rearSpringMotionRatio_mmpmm'  dataShape=Scalar  idxSource=Input  idxRow=1  idxCol=1
      settings: SourceProductName=Raptor
  raptor_data_read4 : Raptor_lib/Data Storage/raptor_data_read  dataName='DATA_frontNonSuspendedMass_kg'  dataShape=Scalar  idxSource=Input  idxRow=1  idxCol=1
      settings: SourceProductName=Raptor
  raptor_data_read5 : Raptor_lib/Data Storage/raptor_data_read  dataName='DATA_frontNonSuspendedMassCGHeight_mm'  dataShape=Scalar  idxSource=Input  idxRow=1  idxCol=1
      settings: SourceProductName=Raptor
  raptor_data_read6 : Raptor_lib/Data Storage/raptor_data_read  dataName='DATA_frontTrack_mm'  dataShape=Scalar  idxSource=Input  idxRow=1  idxCol=1
      settings: SourceProductName=Raptor
  raptor_data_read7 : Raptor_lib/Data Storage/raptor_data_read  dataName='DATA_rearNonSuspendedMass_kg'  dataShape=Scalar  idxSource=Input  idxRow=1  idxCol=1
      settings: SourceProductName=Raptor
  raptor_data_read8 : Raptor_lib/Data Storage/raptor_data_read  dataName='DATA_rearNonSuspendedMassCGHeight_mm'  dataShape=Scalar  idxSource=Input  idxRow=1  idxCol=1
      settings: SourceProductName=Raptor
  raptor_data_read9 : Raptor_lib/Data Storage/raptor_data_read  dataName='DATA_suspendedMass_kg'  dataShape=Scalar  idxSource=Input  idxRow=1  idxCol=1
      settings: SourceProductName=Raptor
  CTRL_dynamicLoadFL_N : Outport
  CTRL_dynamicLoadFR_N : Outport  Port=2
  CTRL_dynamicLoadRL_N : Outport  Port=3
  CTRL_dynamicLoadRR_N : Outport  Port=4
  wires:
  raptor_data_read19/1 -> fz/15(rearTrack)
  raptor_data_read21/1 -> fz/23(wheelBase)
  raptor_data_read25/1 -> fz/27(downForceDistribution)
  raptor_data_read14/1 -> fz/18(rearTireStiffness)
  raptor_data_read3/1 -> fz/4(rearSpringMotionRatio)
  raptor_data_read2/1 -> fz/2(frontSpringMotionRatio)
  raptor_data_read20/1 -> fz/22(suspendedMassCGCoordinatesZ)
  raptor_data_read6/1 -> fz/8(frontTrack)
  raptor_data_read10/1 -> fz/10(suspendedMassWeightDistribution)
  raptor_data_read13/1 -> fz/12(frontTireStiffness)
  raptor_data_read11/1 -> fz/11(frontRollCenterHeight)
  MM5_ay/1 -> fz/6(MM5_ay)
  raptor_data_read9/1 -> fz/9(suspendedMass)
  raptor_data_read7/1 -> fz/19(rearNonSuspendedMass)
  raptor_data_read16/1 -> fz/14(frontARBMotionRatio)
  raptor_data_read23/1 -> fz/25(totalMassDistribution)
  raptor_data_read24/1 -> fz/26(totalDownForce)
  raptor_data_read18/1 -> fz/17(rearARBMotionRatio)
  raptor_data_read12/1 -> fz/21(rearRollCenterHeight)
  raptor_data_read15/1 -> fz/16(rearARBStiffness)
  raptor_data_read26/1 -> fz/28(gravity)
  raptor_data_read22/1 -> fz/24(totalMass)
  raptor_data_read8/1 -> fz/20(rearNonSuspendedMassCGHeight)
  raptor_data_read/1 -> fz/1(frontSpringStiffness)
  raptor_data_read17/1 -> fz/13(frontARBStiffness)
  raptor_data_read1/1 -> fz/3(rearSpringStiffness)
  raptor_data_read5/1 -> fz/7(frontNonSuspendedMassCGHeight)
  raptor_data_read4/1 -> fz/5(frontNonSuspendedMass)
  fz/1(dynamicLoadFL) -> CTRL_dynamicLoadFL_N/1
  fz/2(dynamicLoadFR) -> CTRL_dynamicLoadFR_N/1
  fz/3(dynamicLoadRL) -> CTRL_dynamicLoadRL_N/1
  fz/4(dynamicLoadRR) -> CTRL_dynamicLoadRR_N/1

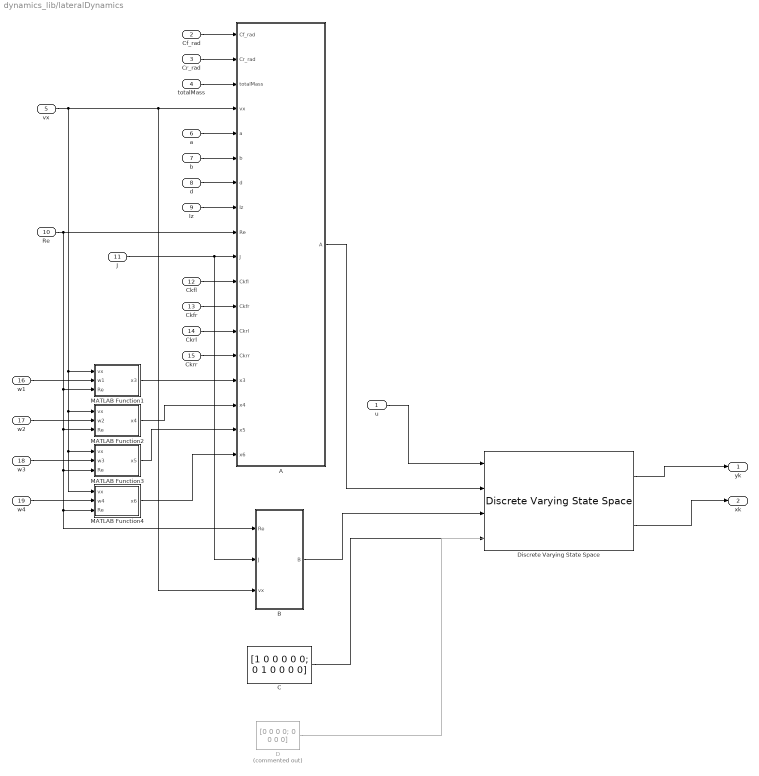
== system dynamics_lib/lateralDynamics ==
  u : Inport
  Cf_rad : Inport  Port=2
  Cr_rad : Inport  Port=3
  totalMass : Inport  Port=4
  vx : Inport  Port=5
  a : Inport  Port=6
  b : Inport  Port=7
  d : Inport  Port=8
  Iz : Inport  Port=9
  Re : Inport  Port=10
  J : Inport  Port=11
  Ckfl : Inport  Port=12
  Ckfr : Inport  Port=13
  Ckrl : Inport  Port=14
  Ckrr : Inport  Port=15
  w1 : Inport  Port=16
  w2 : Inport  Port=17
  w3 : Inport  Port=18
  w4 : Inport  Port=19
  A : MATLAB Function  TreatAsAtomicUnit=on
  B : MATLAB Function  TreatAsAtomicUnit=on
  C : Constant  Value=[1 0 0 0 0 0; 0 1 0 0 0 0]  VectorParams1D=off
  D : Constant  Commented=on  Value=[0 0 0 0; 0 0 0 0]  VectorParams1D=off
  Discrete Varying State Space : cstblocks/Linear Parameter Varying/Discrete Varying State Space  x0=0  Ts=-1  OutputX=on  OutputDX=off  Feedthrough=off
  MATLAB Function1 : MATLAB Function  TreatAsAtomicUnit=on
  MATLAB Function2 : MATLAB Function  TreatAsAtomicUnit=on
  MATLAB Function3 : MATLAB Function  TreatAsAtomicUnit=on
  MATLAB Function4 : MATLAB Function  TreatAsAtomicUnit=on
  yk : Outport
  xk : Outport  Port=2
  wires:
  u/1 -> Discrete Varying State Space/1
  Discrete Varying State Space/1 -> yk/1
  A/1(A) -> Discrete Varying State Space/2
  Discrete Varying State Space/2 -> xk/1
  MATLAB Function1/1(x3) -> A/15(x3)
  MATLAB Function2/1(x4) -> A/16(x4)
  MATLAB Function3/1(x5) -> A/17(x5)
  MATLAB Function4/1(x6) -> A/18(x6)
  Cf_rad/1 -> A/1(Cf_rad)
  Cr_rad/1 -> A/2(Cr_rad)
  totalMass/1 -> A/3(totalMass)
  vx/1 -> MATLAB Function4/1(vx), MATLAB Function3/1(vx), MATLAB Function2/1(vx), MATLAB Function1/1(vx), B/3(vx), A/4(vx)
  J/1 -> B/2(J), A/10(J)
  Iz/1 -> A/8(Iz)
  Re/1 -> B/1(Re), MATLAB Function4/3(Re), MATLAB Function3/3(Re), MATLAB Function2/3(Re), MATLAB Function1/3(Re), A/9(Re)
  d/1 -> A/7(d)
  b/1 -> A/6(b)
  a/1 -> A/5(a)
  Ckrr/1 -> A/14(Ckrr)
  Ckrl/1 -> A/13(Ckrl)
  Ckfr/1 -> A/12(Ckfr)
  Ckfl/1 -> A/11(Ckfl)
  w1/1 -> MATLAB Function1/2(w1)
  w2/1 -> MATLAB Function2/2(w2)
  w4/1 -> MATLAB Function4/2(w4)
  w3/1 -> MATLAB Function3/2(w3)
  B/1(B) -> Discrete Varying State Space/3
  C/1 -> Discrete Varying State Space/4
  D/1 -> ?

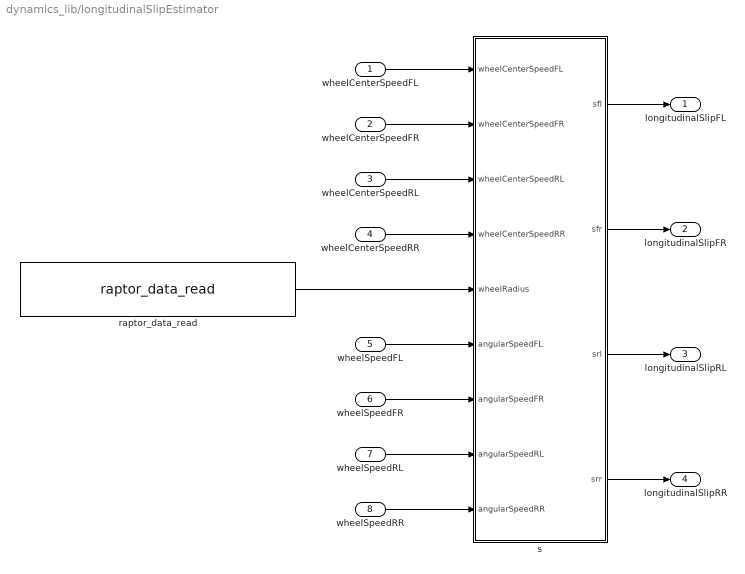
== system dynamics_lib/longitudinalSlipEstimator ==
  wheelCenterSpeedFL : Inport
  wheelCenterSpeedFR : Inport  Port=2
  wheelCenterSpeedRL : Inport  Port=3
  wheelCenterSpeedRR : Inport  Port=4
  wheelSpeedFL : Inport  Port=5
  wheelSpeedFR : Inport  Port=6
  wheelSpeedRL : Inport  Port=7
  wheelSpeedRR : Inport  Port=8
  raptor_data_read : Raptor_lib/Data Storage/raptor_data_read  dataName='DATA_unloadedWheelRadius_m'  dataShape=Scalar  idxSource=Input  idxRow=1  idxCol=1
      settings: SourceProductName=Raptor
  s : MATLAB Function  TreatAsAtomicUnit=on
  longitudinalSlipFL : Outport
  longitudinalSlipFR : Outport  Port=2
  longitudinalSlipRL : Outport  Port=3
  longitudinalSlipRR : Outport  Port=4
  wires:
  s/1(sfl) -> longitudinalSlipFL/1
  s/4(srr) -> longitudinalSlipRR/1
  s/3(srl) -> longitudinalSlipRL/1
  s/2(sfr) -> longitudinalSlipFR/1
  wheelCenterSpeedFL/1 -> s/1(wheelCenterSpeedFL)
  wheelCenterSpeedFR/1 -> s/2(wheelCenterSpeedFR)
  wheelCenterSpeedRL/1 -> s/3(wheelCenterSpeedRL)
  wheelCenterSpeedRR/1 -> s/4(wheelCenterSpeedRR)
  raptor_data_read/1 -> s/5(wheelRadius)
  wheelSpeedRR/1 -> s/9(angularSpeedRR)
  wheelSpeedFL/1 -> s/6(angularSpeedFL)
  wheelSpeedRL/1 -> s/8(angularSpeedRL)
  wheelSpeedFR/1 -> s/7(angularSpeedFR)

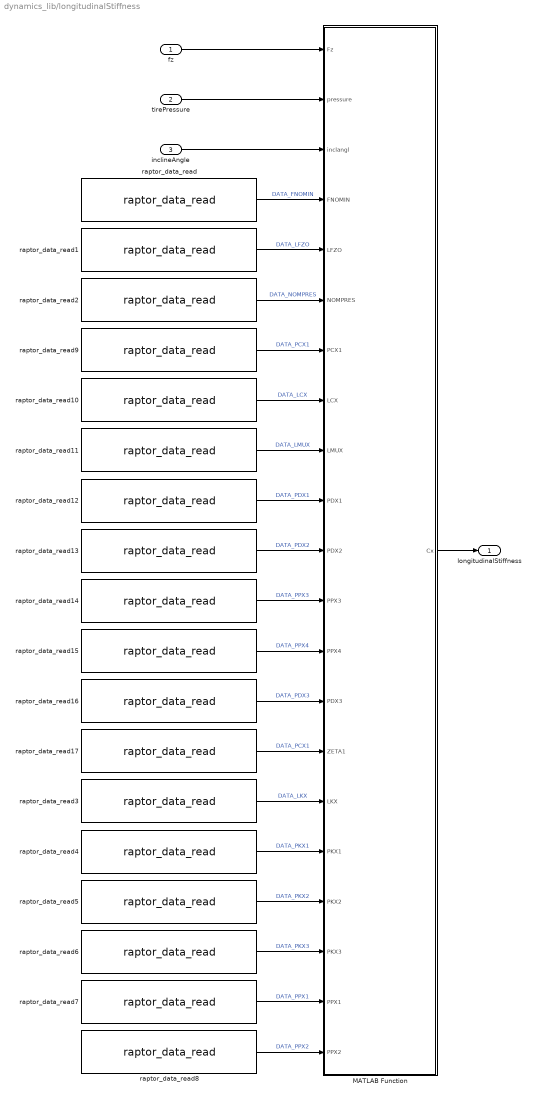
== system dynamics_lib/longitudinalStiffness ==
  fz : Inport
  tirePressure : Inport  Port=2
  inclineAngle : Inport  Port=3
  MATLAB Function : MATLAB Function  TreatAsAtomicUnit=on
  raptor_data_read : Raptor_lib/Data Storage/raptor_data_read  dataName='DATA_FNOMIN_LS'  dataShape=Scalar  idxSource=Input  idxRow=1  idxCol=1
      settings: SourceProductName=Raptor
  raptor_data_read1 : Raptor_lib/Data Storage/raptor_data_read  dataName='DATA_LFZO'  dataShape=Scalar  idxSource=Input  idxRow=1  idxCol=1
      settings: SourceProductName=Raptor
  raptor_data_read10 : Raptor_lib/Data Storage/raptor_data_read  dataName='DATA_LCX'  dataShape=Scalar  idxSource=Input  idxRow=1  idxCol=1
      settings: SourceProductName=Raptor
  raptor_data_read11 : Raptor_lib/Data Storage/raptor_data_read  dataName='DATA_LMUX'  dataShape=Scalar  idxSource=Input  idxRow=1  idxCol=1
      settings: SourceProductName=Raptor
  raptor_data_read12 : Raptor_lib/Data Storage/raptor_data_read  dataName='DATA_PDX1'  dataShape=Scalar  idxSource=Input  idxRow=1  idxCol=1
      settings: SourceProductName=Raptor
  raptor_data_read13 : Raptor_lib/Data Storage/raptor_data_read  dataName='DATA_PDX2'  dataShape=Scalar  idxSource=Input  idxRow=1  idxCol=1
      settings: SourceProductName=Raptor
  raptor_data_read14 : Raptor_lib/Data Storage/raptor_data_read  dataName='DATA_PPX3'  dataShape=Scalar  idxSource=Input  idxRow=1  idxCol=1
      settings: SourceProductName=Raptor
  raptor_data_read15 : Raptor_lib/Data Storage/raptor_data_read  dataName='DATA_PPX4'  dataShape=Scalar  idxSource=Input  idxRow=1  idxCol=1
      settings: SourceProductName=Raptor
  raptor_data_read16 : Raptor_lib/Data Storage/raptor_data_read  dataName='DATA_PDX3'  dataShape=Scalar  idxSource=Input  idxRow=1  idxCol=1
      settings: SourceProductName=Raptor
  raptor_data_read17 : Raptor_lib/Data Storage/raptor_data_read  dataName='DATA_ZETA1'  dataShape=Scalar  idxSource=Input  idxRow=1  idxCol=1
      settings: SourceProductName=Raptor
  raptor_data_read2 : Raptor_lib/Data Storage/raptor_data_read  dataName='DATA_NOMPRES_LS'  dataShape=Scalar  idxSource=Input  idxRow=1  idxCol=1
      settings: SourceProductName=Raptor
  raptor_data_read3 : Raptor_lib/Data Storage/raptor_data_read  dataName='DATA_LKX'  dataShape=Scalar  idxSource=Input  idxRow=1  idxCol=1
      settings: SourceProductName=Raptor
  raptor_data_read4 : Raptor_lib/Data Storage/raptor_data_read  dataName='DATA_PKX1'  dataShape=Scalar  idxSource=Input  idxRow=1  idxCol=1
      settings: SourceProductName=Raptor
  raptor_data_read5 : Raptor_lib/Data Storage/raptor_data_read  dataName='DATA_PKX2'  dataShape=Scalar  idxSource=Input  idxRow=1  idxCol=1
      settings: SourceProductName=Raptor
  raptor_data_read6 : Raptor_lib/Data Storage/raptor_data_read  dataName='DATA_PKX3'  dataShape=Scalar  idxSource=Input  idxRow=1  idxCol=1
      settings: SourceProductName=Raptor
  raptor_data_read7 : Raptor_lib/Data Storage/raptor_data_read  dataName='DATA_PPX1'  dataShape=Scalar  idxSource=Input  idxRow=1  idxCol=1
      settings: SourceProductName=Raptor
  raptor_data_read8 : Raptor_lib/Data Storage/raptor_data_read  dataName='DATA_PPX2'  dataShape=Scalar  idxSource=Input  idxRow=1  idxCol=1
      settings: SourceProductName=Raptor
  raptor_data_read9 : Raptor_lib/Data Storage/raptor_data_read  dataName='DATA_PCX1'  dataShape=Scalar  idxSource=Input  idxRow=1  idxCol=1
      settings: SourceProductName=Raptor
  longitudinalStiffness : Outport
  wires:
  raptor_data_read/1 -> MATLAB Function/4(FNOMIN)  "DATA_FNOMIN"
  raptor_data_read1/1 -> MATLAB Function/5(LFZO)  "DATA_LFZO"
  raptor_data_read2/1 -> MATLAB Function/6(NOMPRES)  "DATA_NOMPRES"
  raptor_data_read3/1 -> MATLAB Function/16(LKX)  "DATA_LKX"
  raptor_data_read5/1 -> MATLAB Function/18(PKX2)  "DATA_PKX2"
  raptor_data_read4/1 -> MATLAB Function/17(PKX1)  "DATA_PKX1"
  raptor_data_read6/1 -> MATLAB Function/19(PKX3)  "DATA_PKX3"
  raptor_data_read7/1 -> MATLAB Function/20(PPX1)  "DATA_PPX1"
  raptor_data_read8/1 -> MATLAB Function/21(PPX2)  "DATA_PPX2"
  fz/1 -> MATLAB Function/1(Fz)
  tirePressure/1 -> MATLAB Function/2(pressure)
  MATLAB Function/1(Cx) -> longitudinalStiffness/1
  inclineAngle/1 -> MATLAB Function/3(inclangl)
  raptor_data_read9/1 -> MATLAB Function/7(PCX1)  "DATA_PCX1"
  raptor_data_read10/1 -> MATLAB Function/8(LCX)  "DATA_LCX"
  raptor_data_read11/1 -> MATLAB Function/9(LMUX)  "DATA_LMUX"
  raptor_data_read12/1 -> MATLAB Function/10(PDX1)  "DATA_PDX1"
  raptor_data_read13/1 -> MATLAB Function/11(PDX2)  "DATA_PDX2"
  raptor_data_read14/1 -> MATLAB Function/12(PPX3)  "DATA_PPX3"
  raptor_data_read15/1 -> MATLAB Function/13(PPX4)  "DATA_PPX4"
  raptor_data_read16/1 -> MATLAB Function/14(PDX3)  "DATA_PDX3"
  raptor_data_read17/1 -> MATLAB Function/15(ZETA1)  "DATA_PCX1"

== system dynamics_lib/rearElWT ==
  MM5_ay : Inport
  CTRL_deltaZ_mm : Inport  Port=2
  CTRL_antiRollRearAxleAndTire_N.m/deg : Inport  Port=3
  CTRL_antiRollTotal_N.m/deg : Inport  Port=4
  raptor_data_read : Raptor_lib/Data Storage/raptor_data_read  dataName='DATA_suspendedMass_kg'  dataShape=Scalar  idxSource=Input  idxRow=1  idxCol=1
      settings: SourceProductName=Raptor
  raptor_data_read1 : Raptor_lib/Data Storage/raptor_data_read  dataName='DATA_rearTrack_mm'  dataShape=Scalar  idxSource=Input  idxRow=1  idxCol=1
      settings: SourceProductName=Raptor
  rearElWT : MATLAB Function  TreatAsAtomicUnit=on
  CTRL_rearElWT_kg : Outport
  wires:
  raptor_data_read/1 -> rearElWT/1(suspendedMass)
  MM5_ay/1 -> rearElWT/2(MM5_ay)
  CTRL_deltaZ_mm/1 -> rearElWT/3(deltaZ)
  raptor_data_read1/1 -> rearElWT/6(rearTrack)
  CTRL_antiRollRearAxleAndTire_N.m/deg/1 -> rearElWT/4(antiRollRearAxleAndTire)
  CTRL_antiRollTotal_N.m/deg/1 -> rearElWT/5(antiRollTotal)
  rearElWT/1(rearElWT) -> CTRL_rearElWT_kg/1

== system dynamics_lib/rearGeoWT ==
  MM5_ay : Inport
  raptor_data_read : Raptor_lib/Data Storage/raptor_data_read  dataName='DATA_suspendedMass_kg'  dataShape=Scalar  idxSource=Input  idxRow=1  idxCol=1
      settings: SourceProductName=Raptor
  raptor_data_read1 : Raptor_lib/Data Storage/raptor_data_read  dataName='DATA_suspendedMassWeightDistribution_pct'  dataShape=Scalar  idxSource=Input  idxRow=1  idxCol=1
      settings: SourceProductName=Raptor
  raptor_data_read2 : Raptor_lib/Data Storage/raptor_data_read  dataName='DATA_rearTrack_mm'  dataShape=Scalar  idxSource=Input  idxRow=1  idxCol=1
      settings: SourceProductName=Raptor
  raptor_data_read3 : Raptor_lib/Data Storage/raptor_data_read  dataName='DATA_rearRollCenterHeight_mm'  dataShape=Scalar  idxSource=Input  idxRow=1  idxCol=1
      settings: SourceProductName=Raptor
  rearGeoWT : MATLAB Function  TreatAsAtomicUnit=on
  CTRL_rearGeoWT_kg : Outport
  wires:
  raptor_data_read1/1 -> rearGeoWT/2(suspendedMassWeightDistribution)
  raptor_data_read/1 -> rearGeoWT/1(suspendedMass)
  MM5_ay/1 -> rearGeoWT/3(MM5_ay)
  raptor_data_read2/1 -> rearGeoWT/5(rearTrack)
  raptor_data_read3/1 -> rearGeoWT/4(rearRollCenterHeight)
  rearGeoWT/1(rearGeoWT) -> CTRL_rearGeoWT_kg/1

== system dynamics_lib/rearNSMWT ==
  MM5_ay : Inport
  raptor_data_read : Raptor_lib/Data Storage/raptor_data_read  dataName='DATA_rearNonSuspendedMass_kg'  dataShape=Scalar  idxSource=Input  idxRow=1  idxCol=1
      settings: SourceProductName=Raptor
  raptor_data_read1 : Raptor_lib/Data Storage/raptor_data_read  dataName='DATA_rearNonSuspendedMassCGHeight_mm'  dataShape=Scalar  idxSource=Input  idxRow=1  idxCol=1
      settings: SourceProductName=Raptor
  raptor_data_read2 : Raptor_lib/Data Storage/raptor_data_read  dataName='DATA_rearTrack_mm'  dataShape=Scalar  idxSource=Input  idxRow=1  idxCol=1
      settings: SourceProductName=Raptor
  rearNSMWT : MATLAB Function  TreatAsAtomicUnit=on
  CTRL_rearNSMWT_kg : Outport
  wires:
  raptor_data_read2/1 -> rearNSMWT/4(rearTrack)
  raptor_data_read1/1 -> rearNSMWT/3(rearNonSuspendedMassCGHeight)
  MM5_ay/1 -> rearNSMWT/2(MM5_ay)
  raptor_data_read/1 -> rearNSMWT/1(rearNonSuspendedMass)
  rearNSMWT/1(rearNSMWT) -> CTRL_rearNSMWT_kg/1

== system dynamics_lib/rearTotalWT ==
  CTRL_rearNSMWT_kg : Inport
  CTRL_rearElWT_kg : Inport  Port=2
  CTRL_rearGeoWT_kg : Inport  Port=3
  rearTotalWT : MATLAB Function  TreatAsAtomicUnit=on
  CTRL_rearTotalWT_kg : Outport
  wires:
  CTRL_rearNSMWT_kg/1 -> rearTotalWT/1(rearNSMWT)
  CTRL_rearElWT_kg/1 -> rearTotalWT/2(rearElWT)
  CTRL_rearGeoWT_kg/1 -> rearTotalWT/3(rearGeoWT)
  rearTotalWT/1(rearTotalWT) -> CTRL_rearTotalWT_kg/1

== system dynamics_lib/rearWheelRate ==
  raptor_data_read : Raptor_lib/Data Storage/raptor_data_read  dataName='DATA_rearSpringStiffness_Npmm'  dataShape=Scalar  idxSource=Input  idxRow=1  idxCol=1
      settings: SourceProductName=Raptor
  raptor_data_read2 : Raptor_lib/Data Storage/raptor_data_read  dataName='DATA_rearSpringMotionRatio_mmpmm'  dataShape=Scalar  idxSource=Input  idxRow=1  idxCol=1
      settings: SourceProductName=Raptor
  rearWheelRate : MATLAB Function  TreatAsAtomicUnit=on
  CTRL_rearWheelRate_N/mm : Outport
  wires:
  raptor_data_read/1 -> rearWheelRate/1(rearSpringStiffness)
  raptor_data_read2/1 -> rearWheelRate/2(rearSpringMotionRatio)
  rearWheelRate/1(rearWheelRate) -> CTRL_rearWheelRate_N/mm/1

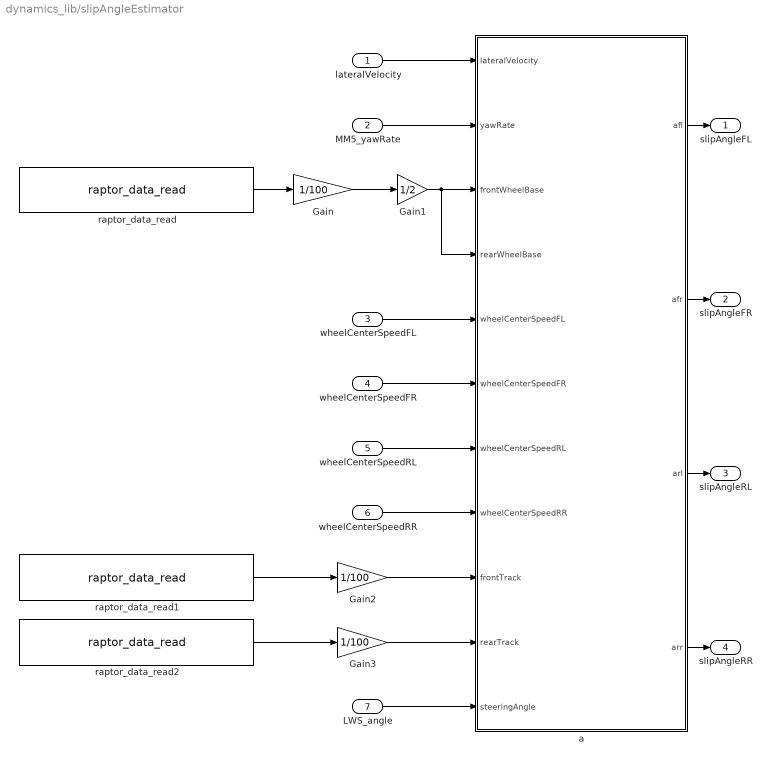
== system dynamics_lib/slipAngleEstimator ==
  lateralVelocity : Inport
  MM5_yawRate : Inport  Port=2
  wheelCenterSpeedFL : Inport  Port=3
  wheelCenterSpeedFR : Inport  Port=4
  wheelCenterSpeedRL : Inport  Port=5
  wheelCenterSpeedRR : Inport  Port=6
  LWS_angle : Inport  Port=7
  Gain : Gain  Gain=1/100
  Gain1 : Gain  Gain=1/2
  Gain2 : Gain  Gain=1/100
  Gain3 : Gain  Gain=1/100
  a : MATLAB Function  TreatAsAtomicUnit=on
  raptor_data_read : Raptor_lib/Data Storage/raptor_data_read  dataName='DATA_wheelBase_mm'  dataShape=Scalar  idxSource=Input  idxRow=1  idxCol=1
      settings: SourceProductName=Raptor
  raptor_data_read1 : Raptor_lib/Data Storage/raptor_data_read  dataName='DATA_frontTrack_mm'  dataShape=Scalar  idxSource=Input  idxRow=1  idxCol=1
      settings: SourceProductName=Raptor
  raptor_data_read2 : Raptor_lib/Data Storage/raptor_data_read  dataName='DATA_rearTrack_mm'  dataShape=Scalar  idxSource=Input  idxRow=1  idxCol=1
      settings: SourceProductName=Raptor
  slipAngleFL : Outport
  slipAngleFR : Outport  Port=2
  slipAngleRL : Outport  Port=3
  slipAngleRR : Outport  Port=4
  wires:
  MM5_yawRate/1 -> a/2(yawRate)
  raptor_data_read/1 -> Gain/1
  Gain/1 -> Gain1/1
  Gain1/1 -> a/4(rearWheelBase), a/3(frontWheelBase)
  wheelCenterSpeedFL/1 -> a/5(wheelCenterSpeedFL)
  raptor_data_read1/1 -> Gain2/1
  raptor_data_read2/1 -> Gain3/1
  LWS_angle/1 -> a/11(steeringAngle)
  a/1(afl) -> slipAngleFL/1
  a/4(arr) -> slipAngleRR/1
  a/3(arl) -> slipAngleRL/1
  a/2(afr) -> slipAngleFR/1
  lateralVelocity/1 -> a/1(lateralVelocity)
  wheelCenterSpeedFR/1 -> a/6(wheelCenterSpeedFR)
  wheelCenterSpeedRL/1 -> a/7(wheelCenterSpeedRL)
  wheelCenterSpeedRR/1 -> a/8(wheelCenterSpeedRR)
  Gain2/1 -> a/9(frontTrack)
  Gain3/1 -> a/10(rearTrack)
